simulink model "HydraulicSystemTesting"  (R2021b)
settings: Solver=FixedStepAuto  StartTime=0.0  StopTime=10.0  FixedStep=1e-3  RelTol=1e-3
undefined symbols (not defined in the file): ABoreSide, ARodSide, beta, FL, k_EV, p_T, pA0, pAMax, pAMin, pB0, pS, VA0, x0, xmax
settings Model: Creator=rrai-HIL  LastModifiedBy=rrai-HIL

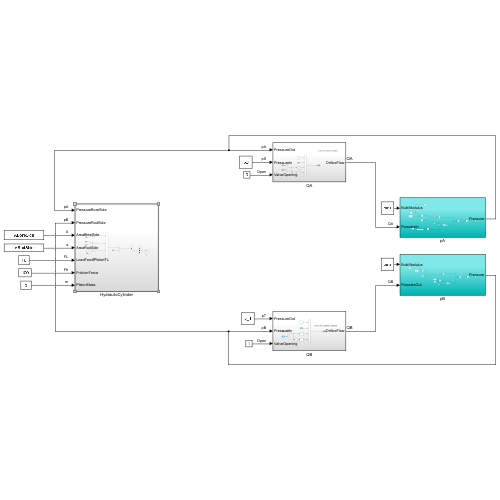
[thumbnail: Simulink's stored preview of the top-level diagram]
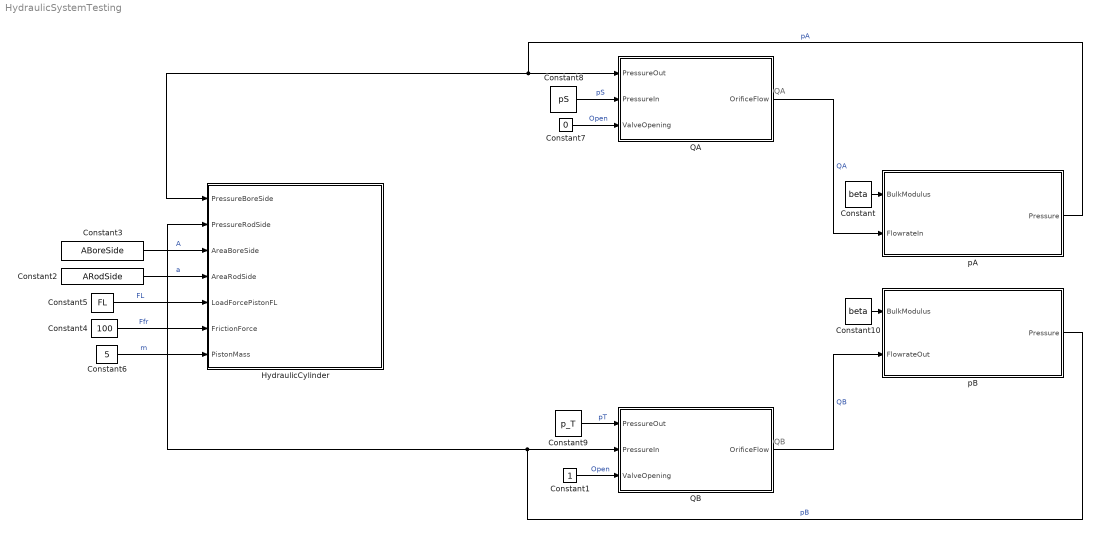
== system HydraulicSystemTesting ==
  note: QA
  note: QB
  Constant : Constant  Value=beta
  Constant1 : Constant
  Constant10 : Constant  Value=beta
  Constant2 : Constant  Value=ARodSide
  Constant3 : Constant  Value=ABoreSide
  Constant4 : Constant  Value=100
  Constant5 : Constant  Value=FL
  Constant6 : Constant  Value=5
  Constant7 : Constant  Value=0
  Constant8 : Constant  Value=pS
  Constant9 : Constant  Value=p_T
  HydraulicCylinder : Subsystem
  QA : Subsystem
  QB : Subsystem
  pA : Subsystem
  pB : Subsystem
  wires:
  pA/1(Pressure) -> QA/1(PressureOut), HydraulicCylinder/1(PressureBoreSide)  "pA"
  pB/1(Pressure) -> QB/2(PressureIn), HydraulicCylinder/2(PressureRodSide)  "pB"
  Constant7/1 -> QA/3(ValveOpening)  "Open"
  Constant1/1 -> QB/3(ValveOpening)  "Open"
  QA/1(OrificeFlow) -> pA/2(FlowrateIn)  "QA"
  Constant3/1 -> HydraulicCylinder/3(AreaBoreSide)  "A"
  Constant2/1 -> HydraulicCylinder/4(AreaRodSide)  "a"
  Constant4/1 -> HydraulicCylinder/6(FrictionForce)  "Ffr"
  Constant5/1 -> HydraulicCylinder/5(LoadForcePistonFL)  "FL"
  Constant6/1 -> HydraulicCylinder/7(PistonMass)  "m"
  Constant/1 -> pA/1(BulkModulus)
  Constant10/1 -> pB/1(BulkModulus)
  QB/1(OrificeFlow) -> pB/2(FlowrateOut)  "QB"
  Constant9/1 -> QB/1(PressureOut)  "pT"
  Constant8/1 -> QA/2(PressureIn)  "pS"

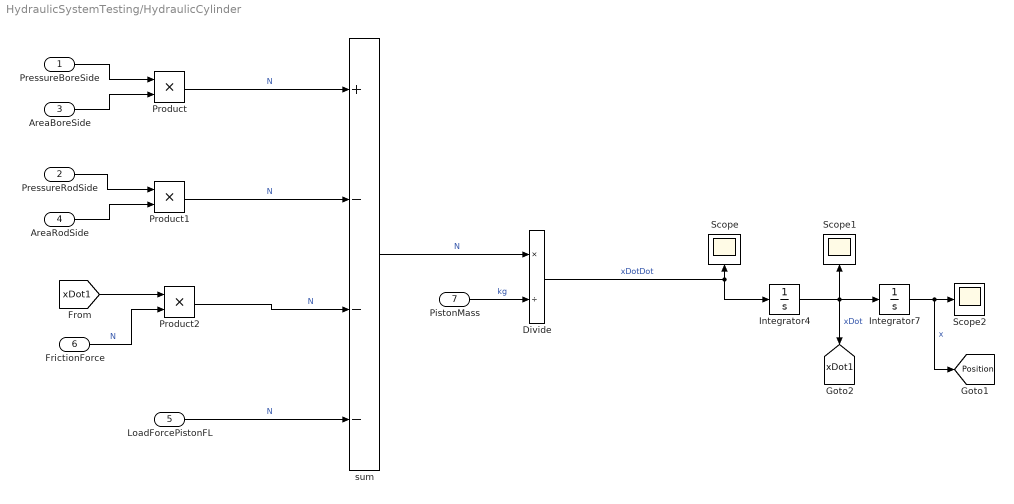
== system HydraulicSystemTesting/HydraulicCylinder ==
  PressureBoreSide : Inport
  PressureRodSide : Inport  Port=2
  AreaBoreSide : Inport  Port=3
  AreaRodSide : Inport  Port=4
  LoadForcePistonFL : Inport  Port=5
  FrictionForce : Inport  Port=6
  PistonMass : Inport  Port=7
  "Divide " : Product  Inputs=*/
  Integrator4 : Integrator  LimitOutput=on  UpperSaturationLimit=1  LowerSaturationLimit=-1
  Integrator7 : Integrator  InitialCondition=x0  LimitOutput=on  UpperSaturationLimit=xmax  LowerSaturationLimit=0
  Product : Product
  Product1 : Product
  Product2 : Product
  Scope : Scope
  Scope1 : Scope
  Scope2 : Scope
  sum : Sum  Inputs=+---
  tag scope: Position=global, xDot1=global
  wires:
  AreaBoreSide/1 -> Product/2
  AreaRodSide/1 -> Product1/2
  PressureRodSide/1 -> Product1/1
  PressureBoreSide/1 -> Product/1
  PistonMass/1 -> "Divide "/2  "kg"
  sum/1 -> "Divide "/1  "N"
  LoadForcePistonFL/1 -> sum/4  "N"
  Product1/1 -> sum/2  "N"
  Product/1 -> sum/1  "N"
  [xDot1] -> Product2/1
  FrictionForce/1 -> Product2/2  "N"
  Product2/1 -> sum/3  "N"
  Integrator7/1 -> [Position], Scope2/1  "x"
  Integrator4/1 -> [xDot1], Scope1/1, Integrator7/1  "xDot"
  "Divide "/1 -> Integrator4/1, Scope/1  "xDotDot"

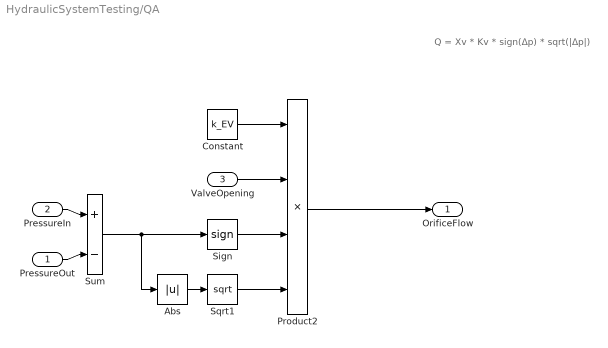
== system HydraulicSystemTesting/QA ==
  note: Q = Xv * Kv * sign(Δp) * sqrt(|Δp|)
  PressureOut : Inport
  PressureIn : Inport  Port=2
  ValveOpening : Inport  Port=3
  Abs : Abs
  Constant : Constant  Value=k_EV
  Product2 : Product  Inputs=4
  Sign : Signum
  Sqrt1 : Sqrt  SaturateOnIntegerOverflow=on
  Sum : Sum  Inputs=+|-
  OrificeFlow : Outport
  wires:
  Constant/1 -> Product2/1
  Abs/1 -> Sqrt1/1
  PressureIn/1 -> Sum/1
  Sum/1 -> Abs/1, Sign/1
  PressureOut/1 -> Sum/2
  Product2/1 -> OrificeFlow/1
  ValveOpening/1 -> Product2/2
  Sqrt1/1 -> Product2/4
  Sign/1 -> Product2/3

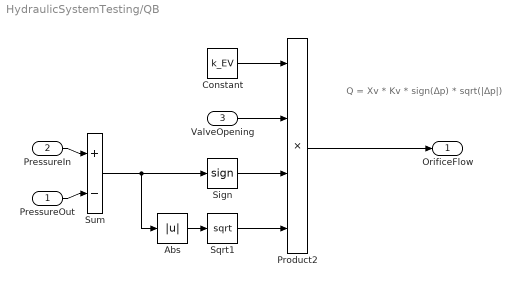
== system HydraulicSystemTesting/QB ==
  note: Q = Xv * Kv * sign(Δp) * sqrt(|Δp|)
  PressureOut : Inport
  PressureIn : Inport  Port=2
  ValveOpening : Inport  Port=3
  Abs : Abs
  Constant : Constant  Value=k_EV
  Product2 : Product  Inputs=4
  Sign : Signum
  Sqrt1 : Sqrt  SaturateOnIntegerOverflow=on
  Sum : Sum  Inputs=+|-
  OrificeFlow : Outport
  wires:
  Constant/1 -> Product2/1
  Abs/1 -> Sqrt1/1
  PressureIn/1 -> Sum/1
  Sum/1 -> Abs/1, Sign/1
  PressureOut/1 -> Sum/2
  Product2/1 -> OrificeFlow/1
  ValveOpening/1 -> Product2/2
  Sqrt1/1 -> Product2/4
  Sign/1 -> Product2/3

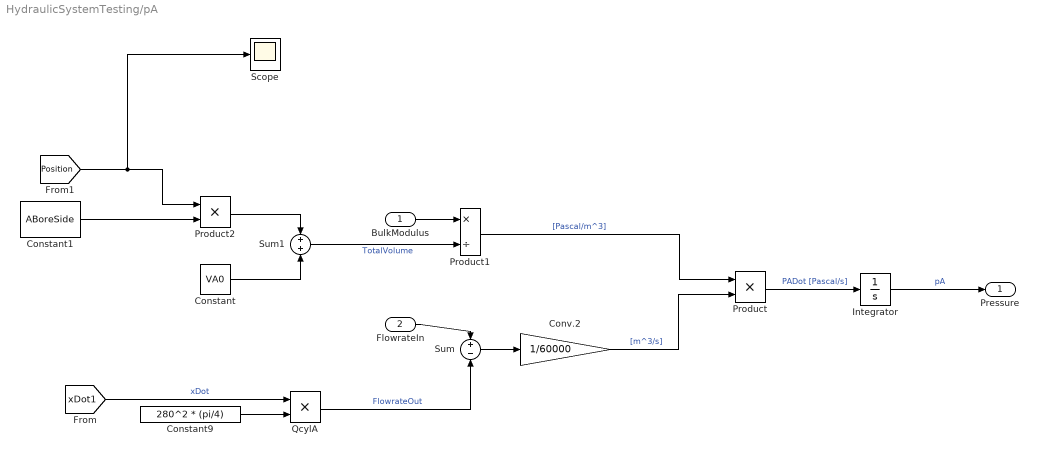
== system HydraulicSystemTesting/pA ==
  BulkModulus : Inport
  FlowrateIn : Inport  Port=2
  Constant : Constant  Value=VA0
  Constant1 : Constant  Value=ABoreSide
  Constant9 : Constant  Value=280^2 * (pi/4)
  Conv.2 : Gain  Gain=1/60000
  Integrator : Integrator  InitialCondition=pA0  LimitOutput=on  UpperSaturationLimit=pAMax  LowerSaturationLimit=pAMin
  Product : Product
  Product1 : Product  Inputs=*/
  Product2 : Product
  QcylA : Product
  Scope : Scope
  Sum : Sum  Inputs=+-
  Sum1 : Sum
  Pressure : Outport
  wires:
  Product1/1 -> Product/1  "[Pascal/m^3]"
  Product/1 -> Integrator/1  "PADot [Pascal/s]"
  Conv.2/1 -> Product/2  "[m^3/s]"
  BulkModulus/1 -> Product1/1
  Sum/1 -> Conv.2/1
  QcylA/1 -> Sum/2  "FlowrateOut"
  FlowrateIn/1 -> Sum/1
  Integrator/1 -> Pressure/1  "pA"
  Sum1/1 -> Product1/2  "TotalVolume"
  Constant/1 -> Sum1/2
  [xDot1] -> QcylA/1  "xDot"
  Constant9/1 -> QcylA/2
  [Position] -> Scope/1, Product2/1
  Constant1/1 -> Product2/2
  Product2/1 -> Sum1/1

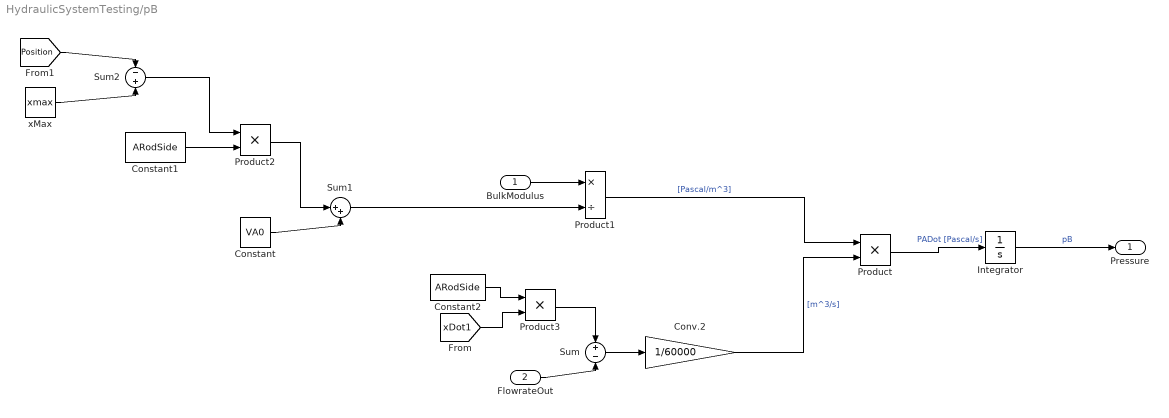
== system HydraulicSystemTesting/pB ==
  BulkModulus : Inport
  FlowrateOut : Inport  Port=2
  Constant : Constant  Value=VA0
  Constant1 : Constant  Value=ARodSide
  Constant2 : Constant  Value=ARodSide
  Conv.2 : Gain  Gain=1/60000
  Integrator : Integrator  InitialCondition=pB0  LimitOutput=on  UpperSaturationLimit=pAMax  LowerSaturationLimit=pAMin
  Product : Product
  Product1 : Product  Inputs=*/
  Product2 : Product
  Product3 : Product
  Sum : Sum  Inputs=+-
  Sum1 : Sum  Inputs=|++
  Sum2 : Sum  Inputs=-+
  xMax : Constant  Value=xmax
  Pressure : Outport
  wires:
  Product1/1 -> Product/1  "[Pascal/m^3]"
  Product/1 -> Integrator/1  "PADot [Pascal/s]"
  Conv.2/1 -> Product/2  "[m^3/s]"
  BulkModulus/1 -> Product1/1
  Sum1/1 -> Product1/2
  Sum/1 -> Conv.2/1
  FlowrateOut/1 -> Sum/2
  Integrator/1 -> Pressure/1  "pB"
  Constant1/1 -> Product2/2
  Product2/1 -> Sum1/1
  Constant/1 -> Sum1/2
  [Position] -> Sum2/1
  xMax/1 -> Sum2/2
  Sum2/1 -> Product2/1
  Constant2/1 -> Product3/1
  [xDot1] -> Product3/2
  Product3/1 -> Sum/1
